simulink model "untitled"  (R2017b)
settings: Solver=VariableStepAuto  StartTime=0.0  StopTime=24  RelTol=1e-3
libraries: checkpacklib x1, dspmtrx3 x1, dspstat3 x1
settings Model: Creator=renato  LastModifiedBy=renato

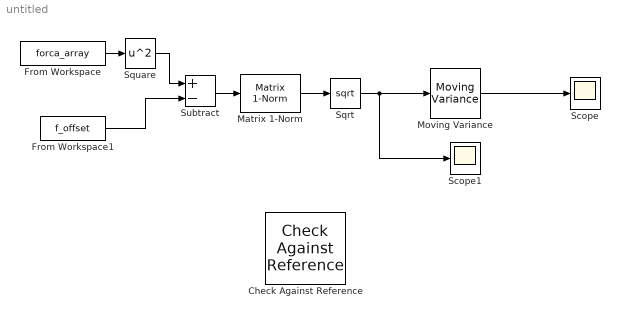
== system untitled ==
  Check Against Reference : checkpacklib/Check Against Reference  InstantiateOnLoad=on  enabled=on  stopWhenAssertionFail=off  export=off  ViewDlgPos=[]  OpenViewOnLoad=off  LaunchViewOnOpen=off  TimeUnits=seconds  EnableReferenceBound=on  AbsTolerance=eps^(1/3)  RelTolerance=0.01  ReferenceTimes=linspace(0,10)  ReferenceAmplitudes=1-exp(-linspace(0,10)/2)
  From Workspace : FromWorkspace  VariableName=forca_array  SampleTime=1
  From Workspace1 : FromWorkspace  VariableName=f_offset  SampleTime=1
  Matrix 1-Norm : dspmtrx3/Matrix  1-Norm  outputDataTypeStr=Inherit: Same as accumulator  outputLastDataTypeStr=Inherit: Same as accumulator  outputMin=[]  outputMax=[]  roundingMode=Floor  overflowMode=off
      settings: SourceProductName=DSP System Toolbox  SourceProductBaseCode=DS
  Moving Variance : dspstat3/Moving Variance  Method=Exponential weighting  SpecifyWindowLength=on  WindowLength=4  ForgettingFactor=0.9  SimulateUsing=Code generation
      settings: SourceProductName=DSP System Toolbox  SourceProductBaseCode=DS
  Scope : Scope
  Scope1 : Scope
  Sqrt : Sqrt  SaturateOnIntegerOverflow=on
  Square : Math  Operator=square  RndMeth=Zero  SaturateOnIntegerOverflow=on
  Subtract : Sum  Inputs=+-
  wires:
  From Workspace1/1 -> Subtract/2
  Moving Variance/1 -> Scope/1
  Matrix 1-Norm/1 -> Sqrt/1
  Sqrt/1 -> Moving Variance/1, Scope1/1
  From Workspace/1 -> Square/1
  Square/1 -> Subtract/1
  Subtract/1 -> Matrix 1-Norm/1
